simulink subsystem "SWPID_Position"  (R2022b)
settings: Solver=VariableStepAuto  StartTime=0.0  StopTime=10.0  RelTol=1e-3
model mask{Kp=1, Ki=1, Kd=0}
  mask prompts: Kp "Simulink:masks:ProportionalP_MP"; Ki "Simulink:masks:IntegralI_MP"; Kd "Simulink:masks:DerivativeD_MP"
libraries: slpidlib x1
settings Model: Creator=gotta  LastModifiedBy=gotta

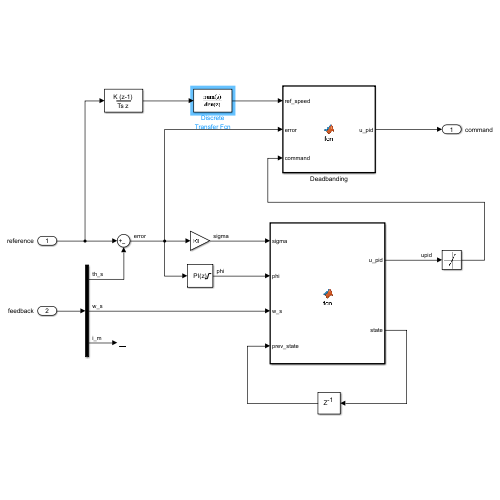
[thumbnail: Simulink's stored preview of the top-level diagram]
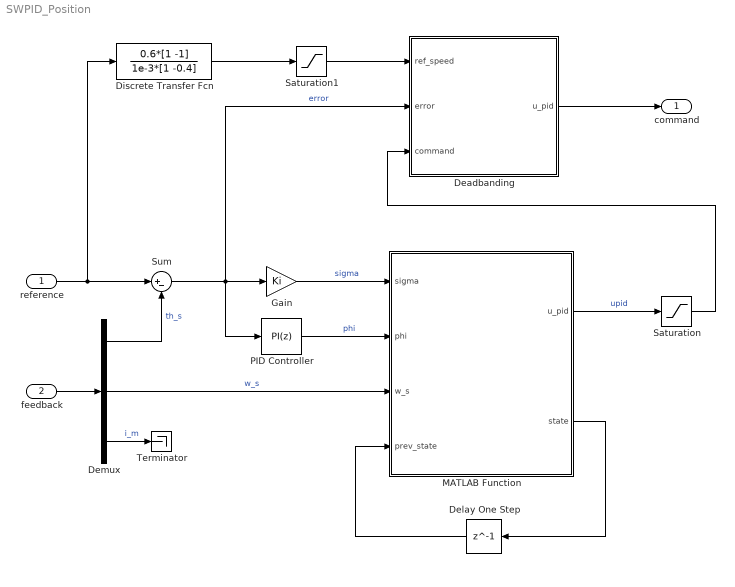
== system SWPID_Position ==
  reference : Inport
  feedback : Inport  Port=2
  Deadbanding : MATLAB Function  TreatAsAtomicUnit=on
  Delay One Step : Delay  DelayLength=1  SampleTime=1e-3
  Demux : Demux  Outputs=3
  Discrete Transfer Fcn : DiscreteTransferFcn  Numerator=0.6*[1 -1]  Denominator=1e-3*[1 -0.4]  SampleTime=1e-3
  Gain : Gain  Gain=Ki
  MATLAB Function : MATLAB Function  TreatAsAtomicUnit=on
  PID Controller : slpidlib/PID Controller  Controller=PI  Form=Ideal  TimeDomain=Discrete-time  UseExternalTs=off  SampleTime=-1  IntegratorMethod=Forward Euler  FilterMethod=Forward Euler  ControllerParametersSource=internal  P=Kp  I=Ki  UseKiTs=off  D=Kd  N=100  UseFilter=on  TunerSelectOption=Transfer Function Based (PID Tuner App)  InitialConditionSource=internal  InitialConditionForIntegrator=0  InitialConditionForFilter=0  DifferentiatorICPrevScaledInput=0  ExternalReset=none  TrackingMode=off  Kt=1  LimitOutput=on  SatLimitsSource=internal  UpperSaturationLimit=5  LowerSaturationLimit=-5  LinearizeAsGain=on  AntiWindupMode=clamping  Kb=1  LimitIntegrator=off  UpperIntegratorSaturationLimit=1  LowerIntegratorSaturationLimit=-1  POutMin=[]  POutMax=[]  IOutMin=[]  IOutMax=[]  DOutMin=[]  DOutMax=[]  NOutMin=[]  NOutMax=[]  SumOutMin=[]  SumOutMax=[]  SaturationOutMin=[]  SaturationOutMax=[]  PParamMin=[]  PParamMax=[]  IParamMin=[]  IParamMax=[]  DParamMin=[]  DParamMax=[]  NParamMin=[]  NParamMax=[]  KbParamMin=[]  KbParamMax=[]  KtParamMin=[]  KtParamMax=[]  KbOutMin=[]  KbOutMax=[]  KtOutMin=[]  KtOutMax=[]  IntegratorOutMin=[]  IntegratorOutMax=[]  FilterOutMin=[]  FilterOutMax=[]  SumI1OutMin=[]  SumI1OutMax=[]  SumI2OutMin=[]  SumI2OutMax=[]  SumI3OutMin=[]  SumI3OutMax=[]  SumI4OutMin=[]  SumI4OutMax=[]  SumDOutMin=[]  SumDOutMax=[]  DifferentiatorOutMin=[]  DifferentiatorOutMax=[]  FilterDiffOutCoefMin=[]  FilterDiffOutCoefMax=[]  ReciprocalOutMin=[]  ReciprocalOutMax=[]  SumDenOutMin=[]  SumDenOutMax=[]  SumNumOutMin=[]  SumNumOutMax=[]  DivideOutMin=[]  DivideOutMax=[]  UdiffTsProdOutMin=[]  UdiffTsProdOutMax=[]  NTsProdOutMin=[]  NTsProdOutMax=[]  UintegralTsProdOutMin=[]  UintegralTsProdOutMax=[]  UngainTsProdOutMin=[]  UngainTsProdOutMax=[]  ClampingZeroOutDataTypeStr=Inherit: Inherit via back propagation  ClampingZeroOutMin=[]  ClampingZeroOutMax=[]  FilterDenConstantOutDataTypeStr=Inherit: Inherit via back propagation  FilterDenConstantOutMin=[]  FilterDenConstantOutMax=[]  PCopyOutDataTypeStr=Inherit: Inherit via back propagation  PCopyOutMin=[]  PCopyOutMax=[]  NCopyOutDataTypeStr=Inherit: Inherit via back propagation  NCopyOutMin=[]  NCopyOutMax=[]  IntegratorContinuousStateAttributes=''  IntegratorStateMustResolveToSignalObject=off  IntegratorRTWStateStorageClass=Auto  FilterContinuousStateAttributes=''  FilterStateMustResolveToSignalObject=off  FilterRTWStateStorageClass=Auto  ParallelPVariant=Passthrough  IdealPVariant=InternalParameters  IVariant=InternalParameters  DVariant=Disabled  IntegratorVariant=Discrete  SatVariant=Enabled  AWVariant=DiscClampingIdeal  PCopyVariant=InternalParamsIdeal  TRVariant=Disabled  FdbkBlocksVariant=Forward  IdealPFdbkVariant=Disabled  SatFdbkVariant=Disabled  DerivativeFilterVariant=Disabled  NVariant=Disabled  NCopyVariant=Disabled_SignalSpec  FilterICVariant=Disabled  IntegratorICVariant=InternalICs  ExternalResetVariant=Disabled  TRSumVariant=Passthrough  SumFdbkVariant=Disabled  SumVariant=Sum_PI  TsampFilterVariant=InternalTs  TsampNgainVariant=Passthrough  TsampIntegralVariant=Passthrough  ExternalSaturationOutDataTypeStr=Inherit: Same as second input
  Saturation : Saturate  UpperLimit=1  LowerLimit=-1
  Saturation1 : Saturate  UpperLimit=1  LowerLimit=-1
  Sum : Sum  Inputs=|+-
  Terminator : Terminator
  command : Outport
  wires:
  feedback/1 -> Demux/1
  Demux/3 -> Terminator/1  "i_m"
  Demux/1 -> Sum/2  "th_s"
  Gain/1 -> MATLAB Function/1(sigma)  "sigma"
  Sum/1 -> Deadbanding/2(error), Gain/1, PID Controller/1  "error"
  Demux/2 -> MATLAB Function/3(w_s)  "w_s"
  MATLAB Function/1(u_pid) -> Saturation/1  "upid"
  PID Controller/1 -> MATLAB Function/2(phi)  "phi"
  MATLAB Function/2(state) -> Delay One Step/1
  Delay One Step/1 -> MATLAB Function/4(prev_state)
  reference/1 -> Discrete Transfer Fcn/1, Sum/1
  Discrete Transfer Fcn/1 -> Saturation1/1
  Saturation/1 -> Deadbanding/3(command)
  Deadbanding/1(u_pid) -> command/1
  Saturation1/1 -> Deadbanding/1(ref_speed)

== matlab function SWPID_Position/Deadbanding ==
  data: ref_speed input; error input; command input; u_pid output
function u_pid = fcn(ref_speed, error, command)

speed_threshold = 0.01;
sensor_threshold = 2*pi/4096;

u_pid = command;

if abs(ref_speed) < speed_threshold && abs(error) <= 2*sensor_threshold
    % reference is fixed and error is within tolerance
    % apply deadbanding
    u_pid = 0;
end

== matlab function SWPID_Position/MATLAB Function ==
  data: sigma input; phi input; w_s input; u_pid output; Kp parameter; Ki parameter; Kd parameter; prev_state input; state output
function [u_pid, state]  = fcn(sigma, phi, w_s, Kp, Ki, Kd, prev_state)

if prev_state == 1 && sigma*phi <= 0
    % transition to overshoot
    phi = -phi;
    state = -1;
elseif prev_state == -1 && w_s*phi >= 0
    % transition to stick-slip
    phi = sigma * Kp / Ki;
    state = 1;
else
    state = prev_state;
end


u_pid = phi - Kd * w_s;
